simulink model "Simulation2DraftWorking"  (R2023a)
settings: Solver=FixedStepDiscrete  StartTime=0.0  StopTime=1  FixedStep=0.01  RelTol=1e-3
undefined symbols (not defined in the file): InputPWM, ticksPerRot, wheelR, WheelSpeed
libraries: mobileRoboticsTrainingLib x7, simulink x2
settings Model: Creator=Boitumelo  LastModifiedBy=ankus
settings DebuggingCC: UnconnectedInputMsg=warning  UnconnectedOutputMsg=warning  UnconnectedLineMsg=warning
settings ModelReferenceCC: EnableRefExpFcnMdlSchedulingChecks=on
settings RTWCC: DLArmComputeVersion=19.05

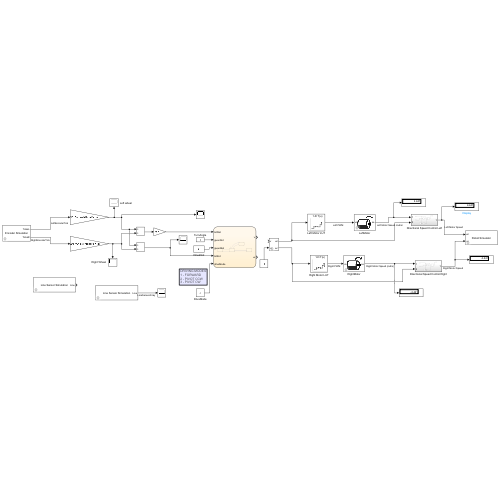
[thumbnail: Simulink's stored preview of the top-level diagram]
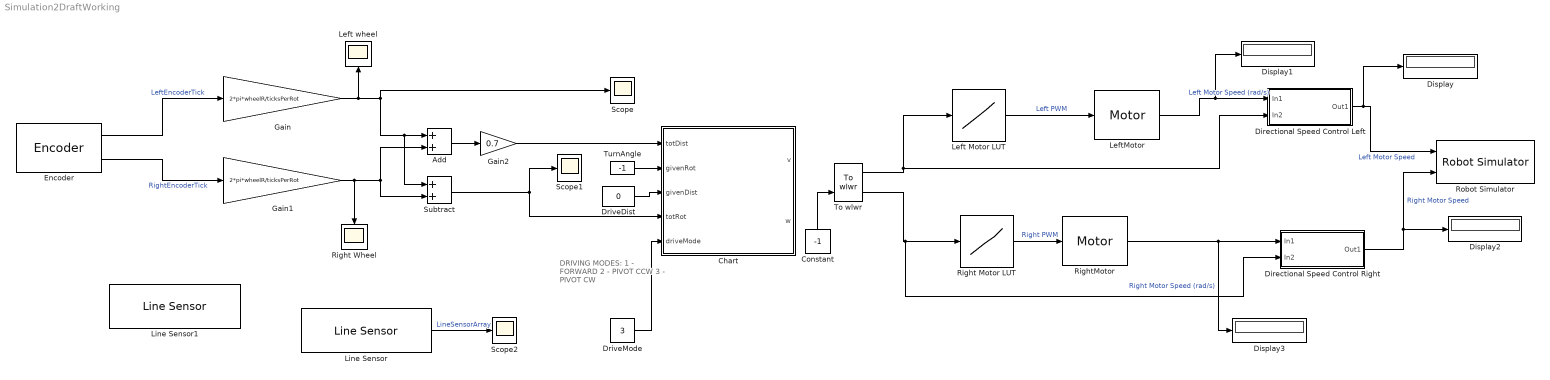
== system Simulation2DraftWorking ==
  note: DRIVING MODES:
      | 1 - FORWARD
      | 2 - PIVOT CCW
      | 3 - PIVOT CW
  Add : Sum
  Chart : Stateflow chart  TreatAsAtomicUnit=on
      settings: PortSchema="{\"entries\":[{\"content\":{\"sides\":[{\"content\":{\"connectorIds\":[\"In4\",\"In3\",\"In1\",\"In5\",\"In2\"]},\"type\":\"ConnectorPlacement.EquallySpacedRectSide\",\"uuid\":\"f0f56214-9b8c-4ddc-aa04-869089de9227\"},{\"content\":{\"connectorIds\":[\"Out1\",\"Out2\"],\"side\":\"RIGHT\"},\"type\":\"ConnectorPlacement.EquallySpacedRectSide\",\"uuid\":\"5b6be25f-9658-4d42-8529-9f359fffebcc\"},{\"content\":{\"side\":\"TOP\"},\"type\":\"ConnectorPlacement.EquallySpacedRectSide\",\"uuid\":\"0183f53a-296c-4206-8b47-a1d28f328d89\"}]},\"type\":\"ConnectorPlacement.EquallySpacedConnector\",\"uuid\":\"a68b37b2-d736-4907-9bf8-ddeeb43f7385\"}],\"packageUris\":[\"http://schema.mathworks.com/mf0/Connector/R2020b\"],\"version\":\"1.0\"}"
  Constant : Constant  Value=-1
  Directional Speed Control Left : Subsystem
  Directional Speed Control Right : Subsystem
  Display{,1..3} (4 alike) : Display
  DriveDist : Constant  Value=0
  DriveMode : Constant  Value=3
  Encoder : mobileRoboticsTrainingLib/Encoder  axleLength=axleLength  wheelR=wheelR  ticksPerRot=ticksPerRot
      settings: SourceProductName=Mobile Robotics Training Library
  Gain : Gain  Gain=2*pi*wheelR/ticksPerRot
  Gain1 : Gain  Gain=2*pi*wheelR/ticksPerRot
  Gain2 : Gain  Gain=0.7
  Left Motor LUT : Lookup_n-D  NumberOfTableDimensions=1  BreakpointsForDimension1=WheelSpeed  Table=InputPWM  InterpMethod=Nearest  ExtrapMethod=Clip  InternalRulePriority=Speed  RndMeth=Simplest
  "Left wheel " : Scope
  LeftMotor : mobileRoboticsTrainingLib/Motor  motorPlant=wheelMotorModel  sensorType=Speed
      settings: SourceProductName=Mobile Robotics Training Library
  Line Sensor : mobileRoboticsTrainingLib/Line Sensor  mapVariable=mapForSim  envVal=1  lineVal=0  sensOff=[0.0643 0.0354; 0.0675 0.005; 0.0675 -0.005; 0.0643 -0.0354]
      settings: SourceProductName=Mobile Robotics Training Library
  Line Sensor1 : mobileRoboticsTrainingLib/Line Sensor  mapVariable=mapForSim  envVal=2850  lineVal=2950  sensOff=[0.01 0]
      settings: SourceProductName=Mobile Robotics Training Library
  Right Motor LUT : Lookup_n-D  NumberOfTableDimensions=1  BreakpointsForDimension1=WheelSpeed  Table=InputPWM  InterpMethod=Nearest  ExtrapMethod=Clip  InternalRulePriority=Speed  RndMeth=Simplest
  "Right Wheel " : Scope
  RightMotor : mobileRoboticsTrainingLib/Motor  motorPlant=wheelMotorModel  sensorType=Speed
      settings: SourceProductName=Mobile Robotics Training Library
  Robot Simulator : mobileRoboticsTrainingLib/Robot Simulator  Priority=99  mapVar=mapForSim  startX=0.5  startY=0.1  startTheta=90  axleLength=axleLength  wheelR=wheelR
  Scope : Scope
  Scope1 : Scope
  Scope2 : Scope
  Subtract : Sum
  To wlwr : mobileRoboticsTrainingLib/To wlwr  axleLength=axleLength  wheelR=wheelR
      link override change parameters: Gain=[1 -axleLength/2; 1 axleLength/2]
  TurnAngle : Constant  Value=-1
  wires:
  Directional Speed Control Left/1(Out1) -> Display/1, Robot Simulator/1  "Left Motor Speed"
  Right Motor LUT/1 -> RightMotor/1  "Right PWM"
  Left Motor LUT/1 -> LeftMotor/1  "Left PWM"
  Encoder/1 -> Gain/1  "LeftEncoderTick"
  Encoder/2 -> Gain1/1  "RightEncoderTick"
  To wlwr/1 -> Directional Speed Control Left/2(In2), Left Motor LUT/1
  To wlwr/2 -> Directional Speed Control Right/2(In2), Right Motor LUT/1
  Line Sensor/1 -> Scope2/1  "LineSensorArray"
  RightMotor/1 -> Display3/1, Directional Speed Control Right/1(In1)  "Right Motor Speed (rad/s)"
  LeftMotor/1 -> Display1/1, Directional Speed Control Left/1(In1)  "Left Motor Speed (rad/s)"
  Directional Speed Control Right/1(Out1) -> Display2/1, Robot Simulator/2  "Right Motor Speed"
  Gain/1 -> "Left wheel "/1, Subtract/1, Add/1, Scope/1
  Gain1/1 -> "Right Wheel "/1, Subtract/2, Add/2
  Add/1 -> Gain2/1
  DriveMode/1 -> Chart/2(driveMode)
  TurnAngle/1 -> Chart/3(givenRot)
  Gain2/1 -> Chart/4(totDist)
  DriveDist/1 -> Chart/1(givenDist)
  Subtract/1 -> Scope1/1, Chart/5(totRot)
  Constant/1 -> To wlwr/2

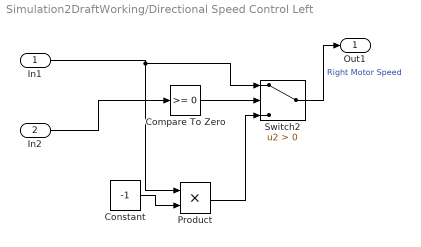
== system Simulation2DraftWorking/Directional Speed Control Left ==
  In1 : Inport
  In2 : Inport  Port=2
  Compare To Zero : simulink/Logic and Bit Operations/Compare To Zero  relop=>=  OutDataTypeStr=boolean
  Constant : Constant  Value=-1
  Product : Product
  Switch2 : Switch  Criteria=u2 > Threshold  SaturateOnIntegerOverflow=off  InputSameDT=off
  Out1 : Outport
  wires:
  Compare To Zero/1 -> Switch2/2
  In1/1 -> Switch2/1, Product/1
  Constant/1 -> Product/2
  Product/1 -> Switch2/3
  In2/1 -> Compare To Zero/1
  Switch2/1 -> Out1/1  "Right Motor Speed"

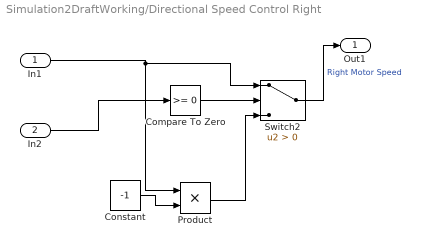
== system Simulation2DraftWorking/Directional Speed Control Right ==
  In1 : Inport
  In2 : Inport  Port=2
  Compare To Zero : simulink/Logic and Bit Operations/Compare To Zero  relop=>=  OutDataTypeStr=boolean
  Constant : Constant  Value=-1
  Product : Product
  Switch2 : Switch  Criteria=u2 > Threshold  SaturateOnIntegerOverflow=off  InputSameDT=off
  Out1 : Outport
  wires:
  Compare To Zero/1 -> Switch2/2
  In1/1 -> Switch2/1, Product/1
  Constant/1 -> Product/2
  Product/1 -> Switch2/3
  In2/1 -> Compare To Zero/1
  Switch2/1 -> Out1/1  "Right Motor Speed"

== stateflow chart Simulation2DraftWorking/Chart ==
  state RotateCW
    entry:
    v = 0;
    w = -0.8;
  state RotateCCW
    entry:
    v = 0;
    w = 500;
  state JustChill
    entry:
    v = 0;
    w=0;
  state MoveForward
    entry:
    v = 0.8;
    w=0;
  JustChill -> RotateCW [order 3] : [driveMode == 3]
  RotateCW -> JustChill : [totRot>=givenRot]
  (default) -> JustChill
  JustChill -> RotateCCW [order 2] : [driveMode == 2]
  JustChill -> MoveForward [order 1] : [driveMode==1]
  MoveForward -> JustChill : [totDist>=givenDist]
  RotateCCW -> JustChill : [totRot>=givenRot]
  data: givenDist input; v output; driveMode input; givenRot input; totDist input; totRot input; w output
